simulink model "gm_biquad_test_v5_old_IP_test"  (R2024b)
settings: Solver=FixedStepDiscrete  StartTime=0.0  StopTime=T  RelTol=1e-12
undefined symbols (not defined in the file or in its folder): a, b, Fs, g, x
libraries: dspsrcs4 x2, dsphdlfiltering2 x1
settings Model: Creator=korvo  LastModifiedBy=korvo
settings OptimizationCC: BlockReduction=off  ConditionallyExecuteInputs=off  DefaultParameterBehavior=Inlined  InheritOutputTypeSmallerThanSingle=on
settings DebuggingCC: AlgebraicLoopMsg=error  ArtificialAlgebraicLoopMsg=error  InheritedTsInSrcMsg=none  SingleTaskRateTransMsg=error  UnconnectedInputMsg=warning  UnconnectedOutputMsg=warning  UnconnectedLineMsg=warning
settings HardwareCC: ProdBitPerPointer=32  ProdBitPerSizeT=32  ProdBitPerPtrDiffT=32  ProdLargestAtomicFloat=None  ProdIntDivRoundTo=Undefined  ProdEndianess=Unspecified  ProdWordSize=32  ProdHWDeviceType=ASIC/FPGA->ASIC/FPGA  TargetBitPerPointer=64  TargetBitPerSizeT=64  TargetBitPerPtrDiffT=64  TargetLongLongMode=on  TargetIntDivRoundTo=Zero  TargetEndianess=LittleEndian  TargetWordSize=64  TargetHWDeviceType=Custom Processor->MATLAB Host Computer  ProdEqTarget=off

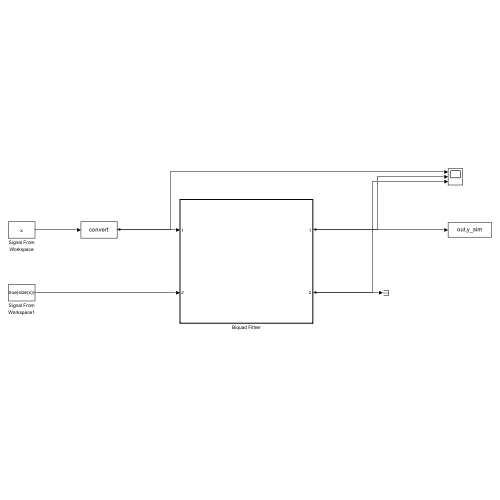
[thumbnail: Simulink's stored preview of the top-level diagram]
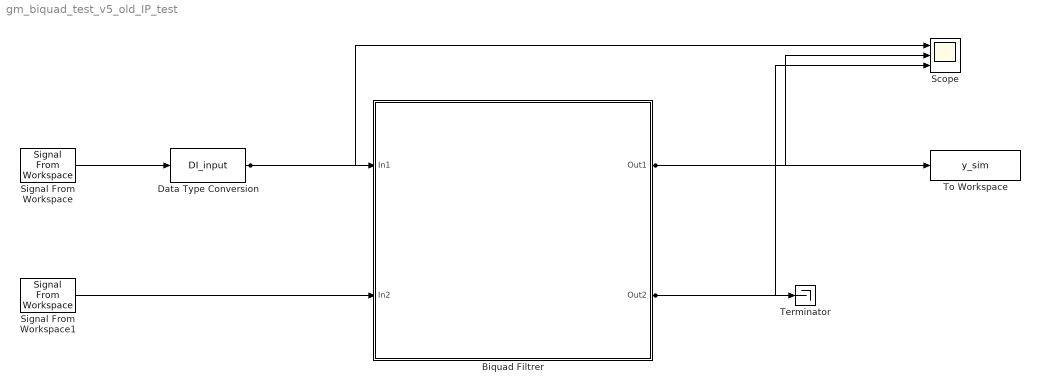
== system gm_biquad_test_v5_old_IP_test ==
  Biquad Filtrer : Subsystem  TreatAsAtomicUnit=on
  Data Type Conversion : DataTypeConversion  OutDataTypeStr=DI_input  SaturateOnIntegerOverflow=off  RndMeth=Floor
  Scope : Scope  NumInputPorts=3
  Signal From Workspace : dspsrcs4/Signal From Workspace  X=x  Ts=1/Fs  nsamps=1  OutputAfterFinalValue=Setting to zero  ignoreOrWarnInputAndFrameLengths=off  OutputFrames=off
  Signal From Workspace1 : dspsrcs4/Signal From Workspace  X=true(size(x))  Ts=1/Fs  nsamps=1  OutputAfterFinalValue=Setting to zero  ignoreOrWarnInputAndFrameLengths=off  OutputFrames=off
  Terminator : Terminator
  To Workspace : ToWorkspace  VariableName=y_sim  SampleTime=-1
      settings: Save2DSignal=2-D array (concatenate along first dimension)
  wires:
  Signal From Workspace1/1 -> Biquad Filtrer/2(In2)
  Data Type Conversion/1 -> Biquad Filtrer/1(In1), Scope/1
  Biquad Filtrer/2(Out2) -> Terminator/1, Scope/3
  Biquad Filtrer/1(Out1) -> To Workspace/1, Scope/2
  Signal From Workspace/1 -> Data Type Conversion/1

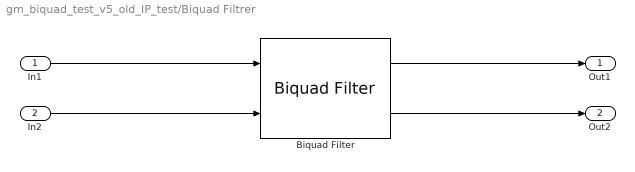
== system gm_biquad_test_v5_old_IP_test/Biquad Filtrer ==
  In1 : Inport
  In2 : Inport  Port=2
  Biquad Filter : dsphdlfiltering2/Biquad Filter  Structure=Direct form II  Numerator=[b ]  Denominator=[ a ]  ScaleValues=[ g]  SimulateUsing=Code generation  roundingMode=Floor  overflowMode=off  NumeratorDataTypeStr=Inherit: Same word length as input  DenominatorDataTypeStr=Inherit: Same word length as input  ScaleValuesDataTypeStr=Inherit: Same word length as input  CoefficientsDataTypeStr=Inherit: Same word length as input
  Out1 : Outport
  Out2 : Outport  Port=2
  wires:
  Biquad Filter/2 -> Out2/1
  In2/1 -> Biquad Filter/2
  Biquad Filter/1 -> Out1/1
  In1/1 -> Biquad Filter/1
